simulink model "ee_loadflow_2bus"  (R2021a)
settings: Solver=VariableStepAuto  StartTime=0.0  StopTime=20  FixedStep=2e-6  RelTol=1e-3  AbsTol=1e-3  EnableMultiTasking=on
libraries: ee_lib x7, fl_lib x6, nesl_utility x1
CloseFcn:
  | try,close(h1_ee_loadflow_2bus),end
  | clear h1_ee_loadflow_2bus
  | 
  | clear simlog_ee_loadflow_2bus
  | clear logsout_ee_loadflow_2bus
Description:
  | 2-Bus Loadflow
settings Model: Creator=The MathWorks, Inc.  LastModifiedBy=dkh20
settings SolverCC: AutoScaleAbsTol=off  AlgebraicLoopSolver=TrustRegion
settings DataIOCC: MaxDataPoints=110000  SaveOutput=off  SignalLogging=off  DSMLogging=off  SaveTime=off  ReturnWorkspaceOutputs=off  SignalLoggingName=logsout_ee_loadflow_ieee9bus
settings OptimizationCC: LifeSpan=inf
settings DebuggingCC: UnderspecifiedInitializationDetection=Classic  MergeDetectMultiDrivingBlocksExec=none  MaxConsecutiveZCsMsg=warning  SFUnexpectedBacktrackingDiag=warning  SFNoUnconditionalDefaultTransitionDiag=warning  SFExecutionAtInitializationDiag=none  SFMachineParentedDataDiag=warning  ArithmeticOperatorsInVariantConditions=warning
settings SFSimCC: SimUseLocalCustomCode=off
settings RTWCC: RTWUseLocalCustomCode=off
settings CodeAppCC: StateflowObjectComments=on
settings GRTTargetCC: TargetLangStandard=C89/C90 (ANSI)
settings ConfigComp: CovMetricSettings=dw  CovSaveCumulativeToWorkspaceVar=on  CovSaveSingleToWorkspaceVar=on  CovExternalEMLEnable=off
settings SimscapeCC: SimscapeNormalizeSystem=off  SimscapeLogType=all  SimscapeLogSimulationStatistics=on  SimscapeLogName=simlog_ee_loadflow_2bus

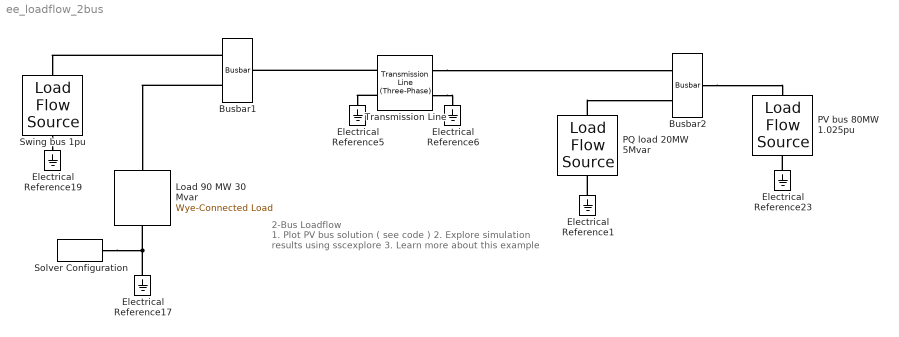
== system ee_loadflow_2bus ==
  note: 2-Bus Loadflow
  note: 1. Plot PV bus solution ( see code )
      | 2. Explore simulation results using sscexplore
      | 3. Learn more about this example
  Busbar1 : ee_lib/Connectors & References/Busbar  Tag="1.000 pu\\n0.00 deg\\n30.4   59.6  -90.0 MW\\n7.5   22.5  -30.0 Mvar"  n_nodes=ee.enum.connectors.busbar_number_of_connections.three  VRated=13.8 kV  freq=60 Hz  show_ps=ee.enum.connectors.busbar_measurement.false
      settings: AttributesFormatString=%<Tag>  SourceProductBaseCode=PS  InternalSimscapePortConfiguration="{\"Bottom\":[],\"Left\":[{\"id\":\"N1\",\"label\":\"~1\",\"type\":\"foundation.electrical.three_phase\"},{\"id\":\"N3\",\"label\":\"~3\",\"type\":\"foundation.electrical.three_phase\"}],\"Right\":[{\"id\":\"N2\",\"label\":\"~2\",\"type\":\"foundation.electrical.three_phase\"}],\"Top\":[]}"
  Busbar2 : ee_lib/Connectors & References/Busbar  Tag="1.025 pu\\n2.51 deg\\n-60.0   80.0  -20.0 MW\\n-25.6   30.6   -5.0 Mvar"  n_nodes=ee.enum.connectors.busbar_number_of_connections.three  VRated=13.8 kV  freq=60 Hz  show_ps=ee.enum.connectors.busbar_measurement.false
      settings: AttributesFormatString=%<Tag>  SourceProductBaseCode=PS  InternalSimscapePortConfiguration="{\"Bottom\":[],\"Left\":[{\"id\":\"N1\",\"label\":\"~1\",\"type\":\"foundation.electrical.three_phase\"},{\"id\":\"N3\",\"label\":\"~3\",\"type\":\"foundation.electrical.three_phase\"}],\"Right\":[{\"id\":\"N2\",\"label\":\"~2\",\"type\":\"foundation.electrical.three_phase\"}],\"Top\":[]}"
  Electrical Reference{1,5..6,17,19,23} (6 alike) : fl_lib/Electrical/Electrical Elements/Electrical Reference
  Load 90 MW 30 Mvar : ee_lib/Passive/RLC Assemblies/Wye-Connected Load  parameterization=2  component_structure=1  component_structure_PQ=4  R=1 Ohm  L=0.001 H  C=1e-6 F  R_parasitic=1e-6 Ohm  G_parasitic=1e-6 1/Ohm  VRated=13.8 kV  FRated=60 Hz  P=90 MW  Qpos=30 MW  Qneg=-100 V*A  Vmag0=230e3 V  Vang0=0 rad  Freq0=60 Hz  R_parasitic_PQ=1e-6 Ohm  G_parasitic_PQ=1e-6*0 1/Ohm  IL_specify=on  IL_priority=High  IL=[ 0 0 0 ] A  IL_nominal_specify=off  IL_nominal_unit=A  IL_nominal_value=1  VC_specify=on  VC_priority=High  VC=[ 0 0 0 ] V  VC_nominal_specify=off  VC_nominal_unit=V  VC_nominal_value=1
      settings: SourceProductBaseCode=PS
  PQ load 20MW 5Mvar : ee_lib/Sources/Load Flow Source  source_type=ee.enum.sources.load_flow_source_type.PQ  v_pu_src=1  active_power_generated=85 MW  active_power_consumed=20 MW  reactive_power_consumed=5 MW  v_pu=1.025  minimum_pu=0.95  phase_search_range=[-30, 30] deg  VRated=13.8 kV  freq=60 Hz  shift_src=0 deg  impedance_option=ee.enum.sources.load_flow_source_impedance.None  SShortCircuit=8000 MW  XR=15  R=0.01 Ohm  L=3.97e-4 H  G_parasitic=0 1/Ohm  I_specify=off  I_priority=None  I=[ 0 0 0 ] A  I_nominal_specify=off  I_nominal_unit=A  I_nominal_value=1  V_impedance_specify=off  V_impedance_priority=None  V_impedance=[ 0 0 0 ] V  V_impedance_nominal_specify=off  V_impedance_nominal_unit=V  V_impedance_nominal_value=1
      settings: SourceProductBaseCode=PS  InternalSimscapePortConfiguration="{\"Bottom\":[],\"Left\":[{\"id\":\"N\",\"label\":\"~\",\"type\":\"foundation.electrical.three_phase\"}],\"Right\":[{\"id\":\"n\",\"label\":\"n\",\"type\":\"foundation.electrical.electrical\"}],\"Top\":[]}"
  PV bus 80MW 1.025pu : ee_lib/Sources/Load Flow Source  source_type=ee.enum.sources.load_flow_source_type.PV  v_pu_src=1  active_power_generated=80 MW  active_power_consumed=0 W  reactive_power_consumed=0 W  v_pu=1.025  minimum_pu=0.95  phase_search_range=[-30, 30] deg  VRated=13.8 kV  freq=60 Hz  shift_src=0 deg  impedance_option=ee.enum.sources.load_flow_source_impedance.XRratio  SShortCircuit=8000 MW  XR=15  R=0.01 Ohm  L=3.97e-4 H  G_parasitic=0 1/Ohm  I_specify=off  I_priority=None  I=[ 0 0 0 ] A  I_nominal_specify=off  I_nominal_unit=A  I_nominal_value=1  V_impedance_specify=off  V_impedance_priority=None  V_impedance=[ 0 0 0 ] V  V_impedance_nominal_specify=off  V_impedance_nominal_unit=V  V_impedance_nominal_value=1
      settings: SourceProductBaseCode=PS  InternalSimscapePortConfiguration="{\"Bottom\":[],\"Left\":[{\"id\":\"N\",\"label\":\"~\",\"type\":\"foundation.electrical.three_phase\"}],\"Right\":[{\"id\":\"n\",\"label\":\"n\",\"type\":\"foundation.electrical.electrical\"}],\"Top\":[]}"
  Solver Configuration : nesl_utility/Solver Configuration  PhysicalDomain=network_engine_domain  SubClassName=solver  LeftPortType=input  RightPortType=generic  Tones=[]  Harmonics=[]  SimulateNoise=off  Profile=off  UseLocalSampling=off  EnableSwitchedLinearOptims=on  FrequencyDomain=off  UseCCode=off  RelTol=0.001  AbsTol=1e-06  MinStep=1e-09  ToWorkspace=off  RevertToSquareIcSolve=off  NumHomotopyIterations=100  PhasorMode=off  PhasorModeNumHarmonics=1  DoDC=off  ResidualTolerance=1e-09  UseLocalSolver=off  LocalSolverChoice=NE_BACKWARD_EULER_ADVANCER  LocalSolverSampleTime=0.001  DoFixedCost=off  MaxNonlinIter=3  MaxModeIter=2  ComputeImpulses=off  ImpulseIterations=2  LinearAlgebra=auto  EquationFormulation=NE_FREQUENCY_TIME_EF  DelaysMemoryBudget=1024  AutomaticFiltering=on  FilteringTimeConstant=0.001  PartitionStorageMethod=AS_NEEDED  PartitionMemoryBudget=1024  PartitionMethod=ROBUST
      settings: SourceProductBaseCode=PW,SS
  Swing bus 1pu : ee_lib/Sources/Load Flow Source  source_type=ee.enum.sources.load_flow_source_type.Swing  v_pu_src=1  active_power_generated=163 MW  active_power_consumed=0 W  reactive_power_consumed=0 W  v_pu=1  minimum_pu=0.95  phase_search_range=[-30, 30] deg  VRated=13.8 kV  freq=60 Hz  shift_src=0 deg  impedance_option=ee.enum.sources.load_flow_source_impedance.None  SShortCircuit=8000 MW  XR=15  R=0.01 Ohm  L=3.97e-4 H  G_parasitic=0 1/Ohm  I_specify=off  I_priority=None  I=[ 0 0 0 ] A  I_nominal_specify=off  I_nominal_unit=A  I_nominal_value=1  V_impedance_specify=off  V_impedance_priority=None  V_impedance=[ 0 0 0 ] V  V_impedance_nominal_specify=off  V_impedance_nominal_unit=V  V_impedance_nominal_value=1
      settings: SourceProductBaseCode=PS  InternalSimscapePortConfiguration="{\"Bottom\":[],\"Left\":[{\"id\":\"N\",\"label\":\"~\",\"type\":\"foundation.electrical.three_phase\"}],\"Right\":[{\"id\":\"n\",\"label\":\"n\",\"type\":\"foundation.electrical.electrical\"}],\"Top\":[]}"
  Transmission Line : ee_lib/Passive/Lines/Transmission Line (Three-Phase)  length=1 km  R=0.02 Ohm/km  L=0.5 mH/km  M=0.1 mH/km  Cl=0.3 uF/km  Cg=0 uF/km  Rm=0 Ohm/km  N=1  R_parasitic=1e-6 Ohm  G_parasitic=1e-6 1/Ohm
      settings: SourceProductBaseCode=PS  InternalSimscapePortConfiguration="{\"Bottom\":[],\"Left\":[{\"id\":\"N1\",\"label\":\"~1\",\"type\":\"foundation.electrical.three_phase\"},{\"id\":\"g1\",\"label\":\"g1\",\"type\":\"foundation.electrical.electrical\"}],\"Right\":[{\"id\":\"N2\",\"label\":\"~2\",\"type\":\"foundation.electrical.three_phase\"},{\"id\":\"g2\",\"label\":\"g2\",\"type\":\"foundation.electrical.electrical\"}],\"Top\":[]}"
  connections:
  Swing bus 1pu/RConn1 -- Electrical Reference19/LConn1
  Transmission Line/LConn2 -- Electrical Reference5/LConn1
  Transmission Line/RConn2 -- Electrical Reference6/LConn1
  Electrical Reference23/LConn1 -- PV bus 80MW 1.025pu/RConn1
  Electrical Reference17/LConn1 -- Load 90 MW 30 Mvar/RConn1 -- Solver Configuration/RConn1
  Transmission Line/LConn1 -- Busbar1/RConn1
  Busbar2/RConn1 -- PV bus 80MW 1.025pu/LConn1
  Transmission Line/RConn1 -- Busbar2/LConn1
  Busbar1/LConn1 -- Swing bus 1pu/LConn1
  Busbar1/LConn2 -- Load 90 MW 30 Mvar/LConn1
  PQ load 20MW 5Mvar/LConn1 -- Busbar2/LConn2
  Electrical Reference1/LConn1 -- PQ load 20MW 5Mvar/RConn1
